simulink model "Simulink_Texto"  (R2025b)
settings: Solver=VariableStepAuto  StartTime=0.0  StopTime=Inf  RelTol=1e-3
libraries: simulink x2, commdigbbndpm3 x2, commchan3 x1
settings Model: Creator=enrique  LastModifiedBy=enrique
settings SolverCC: AlgebraicLoopSolver=TrustRegion
settings DebuggingCC: UnconnectedInputMsg=warning  UnconnectedOutputMsg=warning  UnconnectedLineMsg=warning
settings ModelReferenceCC: EnableRefExpFcnMdlSchedulingChecks=on
settings SFSimCC: CustomCodeUndefinedFunction=UseInterfaceOnly
settings RTWCC: GPUComputeCapability=3.5  DLArmComputeVersion=19.05

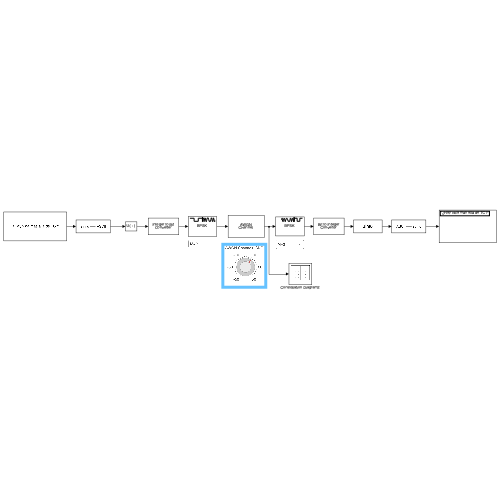
[thumbnail: Simulink's stored preview of the top-level diagram]
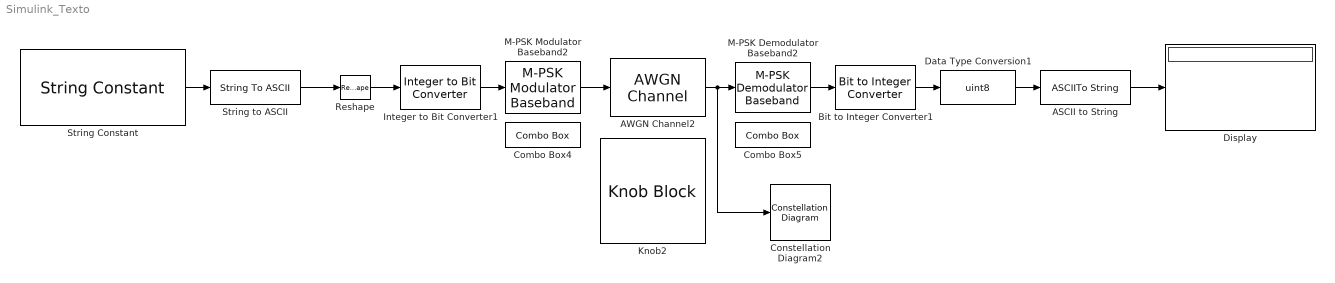
== system Simulink_Texto ==
  ASCII to String : ASCIIToString
  AWGN Channel2 : commchan3/AWGN Channel  LegacyMode=on  NoiseMethod="Signal to noise ratio  (SNR)"  noiseMode="Signal to noise ratio  (SNR)"  EbNo=67  EsNo=10  SNR=12.32153828938802  BitsPerSymbol=1  SignalPower=1  SpecifySymbolPeriod=off  SamplesPerSymbol=1  SymbolPeriod=1  VarianceSource=Parameter  Variance=1  RandomStream=Global stream  Seed=67  SimulateUsing=Code generation
  Bit to Integer Converter1 : simulink/Logic and Bit Operations/Bit to Integer Converter  nbits=8  bitOrder=MSB first  signedOutputValues=Unsigned  outDtype=Inherit via internal rule  outDtypeSigned=Inherit via internal rule
  Combo Box4 : ComboBox  LabelPosition=Hide  SelectedLabel=M=2
  Combo Box5 : ComboBox  LabelPosition=Hide  SelectedLabel=M=2
  Constellation Diagram2 : ConstellationDiagram  WindowPosition=[1638.000000,865.000000,710.000000,481.000000,]  Visible=on  ScopeFrameLocation=window  ReferenceConstellation=BPSK  XLimits=[-1.7976 1.7946]  YLimits=[-1.7976 1.7946]  AxesLimits=[-1.7976 1.7946]  DefaultConfigurationName=comm.scopes.ConstellationDiagramBlockCfg
  Data Type Conversion1 : DataTypeConversion  OutDataTypeStr=uint8  SaturateOnIntegerOverflow=off  RndMeth=Floor
  Display : Display
  Integer to Bit Converter1 : simulink/Logic and Bit Operations/Integer to Bit Converter  nbits=8  signedInputValues=Unsigned  bitOrder=MSB first  outDtype=Inherit via internal rule
  Knob2 : KnobBlock  ScaleMin=-50  ScaleMax=50
  M-PSK Demodulator Baseband2 : commdigbbndpm3/M-PSK Demodulator Baseband  M=2  OutType=Bit  DecType=Hard decision  VarSource=Dialog  Variance=1  Dec=Gray  Mapping=[0:7]  Ph=0  outDtype1=Inherit via internal rule  outDtype2=Inherit via internal rule  derotateFactorWordLen=16  derotateFactorDataTypeStr=Inherit: Same word length as input  derotateFactorLastDataTypeStr=Inherit: Same word length as input
  M-PSK Modulator Baseband2 : commdigbbndpm3/M-PSK Modulator Baseband  M=2  InType=Bit  Enc=Gray  Mapping=[0:7]  Ph=0  outDtype=double  outWordLen=16  outUDDataType=sfix(16)  outFracLenMode=Best precision  outFracLen=15  outDataTypeStr=double  outLastDataTypeStr=double
  Reshape : Reshape
  String Constant : StringConstant  String="\"¿Hay vida más allá de TC?\""
  String to ASCII : StringToASCII  OutputVectorSize=16*3
  wires:
  M-PSK Demodulator Baseband2/1 -> Bit to Integer Converter1/1
  Integer to Bit Converter1/1 -> M-PSK Modulator Baseband2/1
  M-PSK Modulator Baseband2/1 -> AWGN Channel2/1
  AWGN Channel2/1 -> M-PSK Demodulator Baseband2/1, Constellation Diagram2/1
  Bit to Integer Converter1/1 -> Data Type Conversion1/1
  Data Type Conversion1/1 -> ASCII to String/1
  Reshape/1 -> Integer to Bit Converter1/1
  ASCII to String/1 -> Display/1
  String to ASCII/1 -> Reshape/1
  String Constant/1 -> String to ASCII/1
